simulink model "Sat_Control"  (R2018b)
settings: Solver=ode4  StartTime=0.0  StopTime=100  FixedStep=0.001  RelTol=1e-3
settings Model: Creator=carlos  LastModifiedBy=carlos

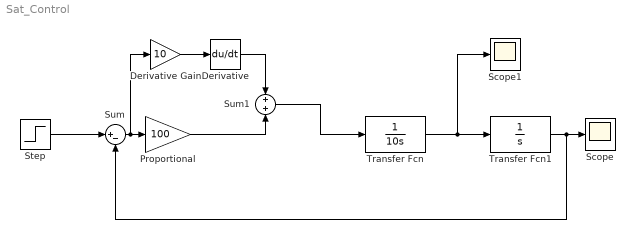
== system Sat_Control ==
  Derivative : Derivative
  "Derivative Gain " : Gain  Gain=10
  "Proportional " : Gain  Gain=100
  Scope : Scope
  Scope1 : Scope
  Step : Step  Time=0  SampleTime=0
  Sum : Sum  Inputs=|+-
  Sum1 : Sum
  Transfer Fcn : TransferFcn  Numerator=1  Denominator=[10 0]
  Transfer Fcn1 : TransferFcn  Numerator=1  Denominator=[1 0]
  wires:
  Transfer Fcn/1 -> Transfer Fcn1/1, Scope1/1
  Transfer Fcn1/1 -> Sum/2, Scope/1
  Step/1 -> Sum/1
  Sum/1 -> "Derivative Gain "/1, "Proportional "/1
  "Derivative Gain "/1 -> Derivative/1
  Derivative/1 -> Sum1/1
  "Proportional "/1 -> Sum1/2
  Sum1/1 -> Transfer Fcn/1
